simulink model "readysecond"  (R2024b)
settings: Solver=VariableStepAuto  StartTime=0.0  StopTime=1  RelTol=1e-3

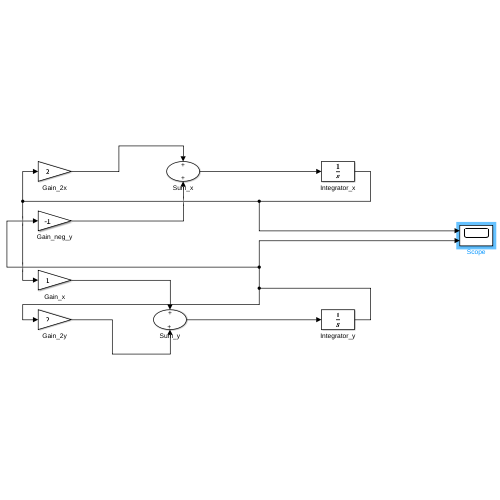
[thumbnail: Simulink's stored preview of the top-level diagram]
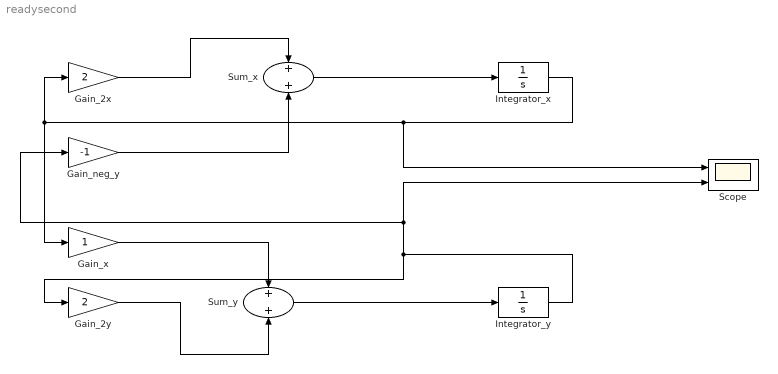
== system readysecond ==
  Gain_2x : Gain  Gain=2
  Gain_2y : Gain  Gain=2
  Gain_neg_y : Gain  Gain=-1
  Gain_x : Gain
  Integrator_x : Integrator  InitialCondition=-1
  Integrator_y : Integrator
  Scope : Scope  NumInputPorts=2
  Sum_x : Sum
  Sum_y : Sum
  wires:
  Sum_x/1 -> Integrator_x/1
  Sum_y/1 -> Integrator_y/1
  Integrator_x/1 -> Gain_2x/1, Gain_x/1, Scope/1
  Integrator_y/1 -> Scope/2, Gain_neg_y/1, Gain_2y/1
  Gain_2x/1 -> Sum_x/1
  Gain_neg_y/1 -> Sum_x/2
  Gain_x/1 -> Sum_y/1
  Gain_2y/1 -> Sum_y/2
